simulink model "Modelo_DINAMICO_2021"  (R2021b)
settings: Solver=VariableStepAuto  StartTime=0.0  StopTime=0.1  MaxStep=1e-5  RelTol=1e-6
values from neighbouring files (symbols this model uses):
  AG0 = 10e-3    (= 0.01)    [Control_5GDL_V2_2021.m]
  beta = 20    [Control_5GDL_V2_2021.m]
  dTSensor = 5e-4    (= 0.0005)    [Control_5GDL_V2_2021.m]
  filterConstant = 30    [Control_5GDL_V2_2021.m]
  noiseSensor = 0.02*1e-3    (= 2e-05)    [Control_5GDL_V2_2021.m]
  z_0 = 17.5e-3    (= 0.0175)    [Control_5GDL_V2_2021.m]
  z_lev = pod.geometry.z_LEV    [Control_5GDL_V2_2021.m]
undefined symbols (not defined in the file or in its folder): initial_conds, pod
libraries: shared6dof x1, simulink_extras x1
settings Model: Creator=emate  LastModifiedBy=Ferran

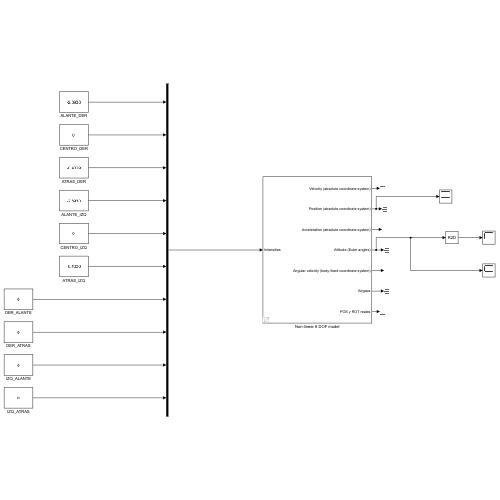
[thumbnail: Simulink's stored preview of the top-level diagram]
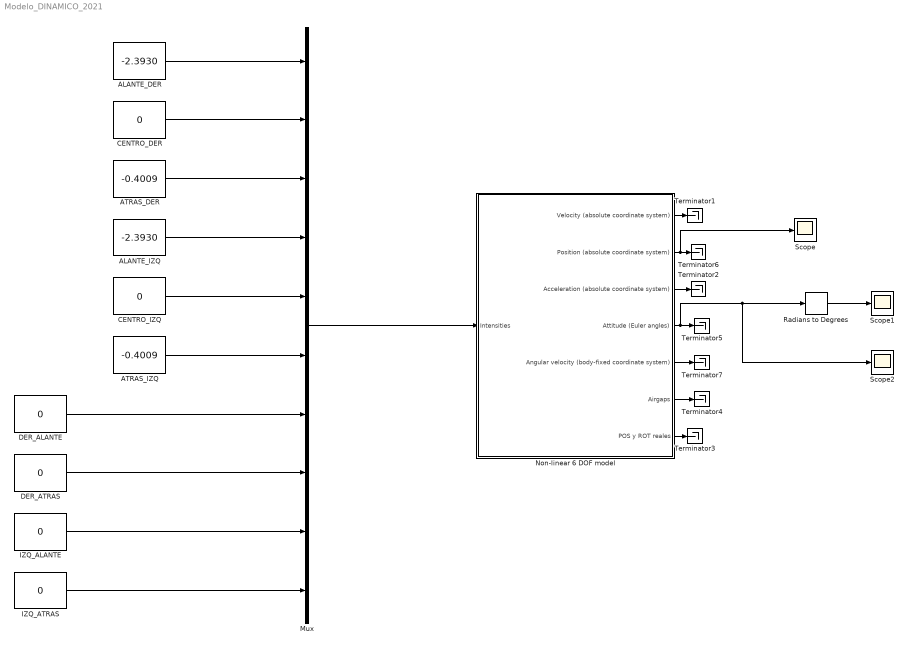
== system Modelo_DINAMICO_2021 ==
  ALANTE_DER : Constant  Value=-2.3930
  ALANTE_IZQ : Constant  Value=-2.3930
  ATRAS_DER : Constant  Value=-0.4009
  ATRAS_IZQ : Constant  Value=-0.4009
  CENTRO_DER : Constant  Value=0
  CENTRO_IZQ : Constant  Value=0
  DER_ALANTE : Constant  Value=0
  DER_ATRAS : Constant  Value=0
  IZQ_ALANTE : Constant  Value=0
  IZQ_ATRAS : Constant  Value=0
  Mux : Mux  Inputs=10
  Non-linear 6 DOF model : Subsystem  AncestorBlock=libH7_6DOF/Non-linear 6 DOF model
  Radians to Degrees : simulink_extras/Transformations/Radians to Degrees
  Scope : Scope
  Scope1 : Scope
  Scope2 : Scope
  Terminator{1..7} (7 alike) : Terminator
  wires:
  Mux/1 -> Non-linear 6 DOF model/1(Intensities)
  ALANTE_DER/1 -> Mux/1
  CENTRO_DER/1 -> Mux/2
  ATRAS_DER/1 -> Mux/3
  ALANTE_IZQ/1 -> Mux/4
  CENTRO_IZQ/1 -> Mux/5
  ATRAS_IZQ/1 -> Mux/6
  DER_ALANTE/1 -> Mux/7
  DER_ATRAS/1 -> Mux/8
  IZQ_ALANTE/1 -> Mux/9
  IZQ_ATRAS/1 -> Mux/10
  Non-linear 6 DOF model/1(Velocity (absolute coordinate system)) -> Terminator1/1
  Non-linear 6 DOF model/3(Acceleration (absolute coordinate system)) -> Terminator2/1
  Non-linear 6 DOF model/7(POS y ROT reales) -> Terminator3/1
  Non-linear 6 DOF model/6(Airgaps) -> Terminator4/1
  Non-linear 6 DOF model/2(Position (absolute coordinate system)) -> Scope/1, Terminator6/1
  Non-linear 6 DOF model/5(Angular velocity (body-fixed coordinate system)) -> Terminator7/1
  Non-linear 6 DOF model/4(Attitude (Euler angles)) -> Radians to Degrees/1, Scope2/1, Terminator5/1
  Radians to Degrees/1 -> Scope1/1

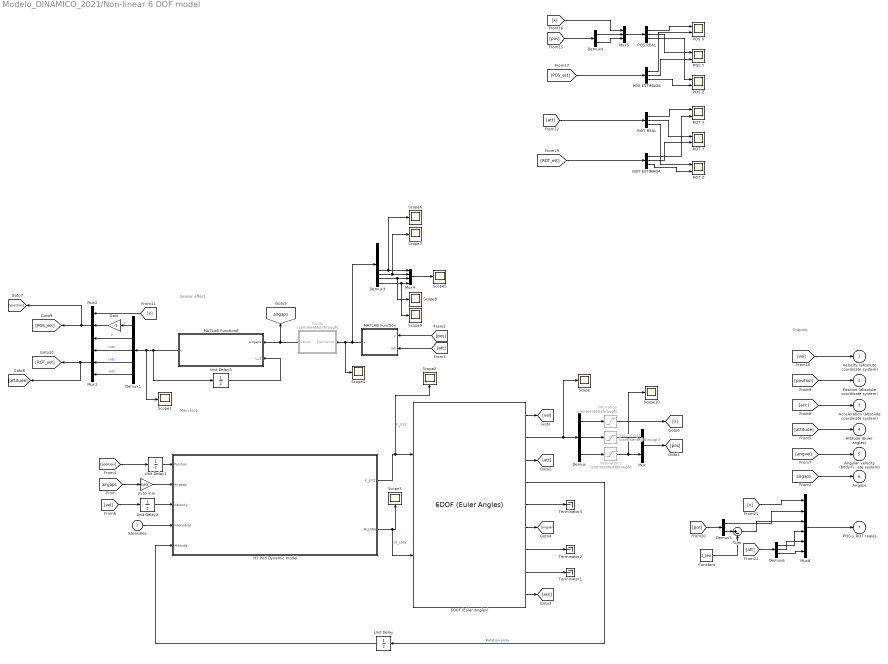
== system Modelo_DINAMICO_2021/Non-linear 6 DOF model ==
  note: Sensor effect
  note: Main loop
  note: Outputs
  Intensities : Inport
  " ROT X" : Scope  NumInputPorts=2
  " ROT Y" : Scope  NumInputPorts=2
  " ROT Z" : Scope  NumInputPorts=2
  6DOF (Euler Angles) : shared6dof/6DOF (Euler Angles)  units=Metric (MKS)  mtype=Fixed  rep=Euler Angles  xme_0=initial_conds.x_0  Vm_0=initial_conds.v_0  eul_0=initial_conds.ang_0  pm_0=initial_conds.w_0  mass_0=pod.mass.mass  mass_e=0.5  mass_f=2.0  inertia=pod.mass.inertia  inertia_e=eye(3)  inertia_f=2*eye(3)  k_quat=1.0  vre_flag=on  abi_flag=on  aMode=0  xme_statename=''  Vm_statename=''  eul_statename=''  quat_statename=''  pm_statename=''  mass_statename=''
      link override Abi: Port=9
      settings: SourceProductBaseCode=AE,PW,DR,MT,UV,VE
  Constant : Constant  Value=z_lev
  Demux : Demux  Outputs=3
  Demux1 : Demux  Outputs=5
  Demux3 : Demux  Outputs=10
  Demux4 : Demux  Outputs=2
  Demux5 : Demux  Outputs=2
  Demux6 : Demux  Outputs=3
  Gain : Gain  Gain=-1
  H7 Pod Dynamic model : Subsystem  AncestorBlock=libH7_6DOF/H7 Pod Dynamic model
      mask Display: image('FBD.png', [0.12 0.12 0.78 0.78]); % Use "Edit Image" on toolstrip to change.
  MATLAB Function : MATLAB Function  TreatAsAtomicUnit=on
  MATLAB Function2 : MATLAB Function  TreatAsAtomicUnit=on
  Mux : Mux  Inputs=2
  Mux1 : Mux  Inputs=3
  Mux2 : Mux  Inputs=3
  Mux4 : Mux
  Mux5 : Mux  Inputs=3
  Mux6 : Mux  Inputs=6
  POS ESTIMADA : Demux  Outputs=3
  POS REAL : Demux  Outputs=3
  POS X : Scope  NumInputPorts=2
  POS Y : Scope  NumInputPorts=2
  POS Z : Scope  NumInputPorts=2
  ROT ESTIMADA : Demux  Outputs=3
  ROT REAL : Demux  Outputs=3
  Ruido : Subsystem  Commented=through
  Saturation : Saturate  Commented=through  UpperLimit=20  LowerLimit=0
  Saturation1 : Saturate  Commented=through  UpperLimit=0.002  LowerLimit=-0.002
  Saturation2 : Saturate  Commented=through  UpperLimit=0.3504  LowerLimit=0.3384
  Scope{,1..10} (11 alike) : Scope
  Sum : Sum  Inputs=|+-
  Terminator1 : Terminator
  Terminator2 : Terminator
  Terminator3 : Terminator
  Unit Delay : UnitDelay  InitialCondition=eye(3,3)  SampleTime=-1  HasFrameUpgradeWarning=on
  Unit Delay1 : UnitDelay  InitialCondition=initial_conds.x_0  SampleTime=-1  HasFrameUpgradeWarning=on
  Unit Delay2 : UnitDelay  InitialCondition=initial_conds.v_0  SampleTime=-1  HasFrameUpgradeWarning=on
  Unit Delay3 : UnitDelay  SampleTime=-1  HasFrameUpgradeWarning=on
  m to mm : Gain  Gain=1e3
  Velocity (absolute coordinate system) : Outport
  Position (absolute coordinate system) : Outport  Port=2
  Acceleration (absolute coordinate system) : Outport  Port=3
  Attitude (Euler angles) : Outport  Port=4
  Angular velocity (body-fixed coordinate system) : Outport  Port=5
  Airgaps : Outport  Port=6
  POS y ROT reales : Outport  Port=7
  tag scope: airgaps=global
  wires:
  Demux1/3 -> Mux1/1  "rotx"
  6DOF (Euler Angles)/8 -> Terminator1/1
  6DOF (Euler Angles)/4 -> Unit Delay/1  "Rotation array"
  6DOF (Euler Angles)/7 -> Terminator2/1
  Unit Delay2/1 -> H7 Pod Dynamic model/3(Velocity)
  Demux/3 -> Saturation2/1
  H7 Pod Dynamic model/2(M_LMN) -> Scope3/1, 6DOF (Euler Angles)/2  "M_LMN"
  H7 Pod Dynamic model/1(F_XYZ) -> Scope2/1, 6DOF (Euler Angles)/1  "F_XYZ"
  Unit Delay/1 -> H7 Pod Dynamic model/5(Attitude)
  6DOF (Euler Angles)/3 -> [att]
  [airgaps] -> m to mm/1
  [position] -> Position (absolute coordinate system)/1
  [vel] -> Velocity (absolute coordinate system)/1
  [airgaps] -> Airgaps/1
  Unit Delay1/1 -> H7 Pod Dynamic model/1(Position)
  [angvel] -> Angular velocity (body-fixed coordinate system)/1
  6DOF (Euler Angles)/6 -> [angvel]
  6DOF (Euler Angles)/2 -> Scope/1, Demux/1
  Demux/2 -> Saturation1/1
  6DOF (Euler Angles)/9 -> [acc]
  [pos] -> MATLAB Function/1(r)
  MATLAB Function2/1(u) -> Unit Delay3/1, Scope1/1, Demux1/1
  [attitude] -> Attitude (Euler angles)/1
  Mux/1 -> [pos]
  Saturation/1 -> [x]
  [att] -> MATLAB Function/2(rot)
  Demux1/2 -> Mux2/3  "z"
  MATLAB Function/1(y) -> Demux3/1, Ruido/1(Estimation), Scope4/1
  Intensities/1 -> H7 Pod Dynamic model/4(Intensities)
  [position] -> Unit Delay1/1
  Unit Delay3/1 -> MATLAB Function2/2(u_1)
  6DOF (Euler Angles)/1 -> [vel]
  Demux1/4 -> Mux1/2  "roty"
  Demux1/5 -> Mux1/3  "rotz"
  [vel] -> Unit Delay2/1
  Demux/1 -> Saturation/1
  Ruido/1(Sensor) -> [airgaps], MATLAB Function2/1(airgaps)
  [x] -> Mux2/1
  Saturation1/1 -> Mux/1
  Demux1/1 -> Gain/1  "y"
  6DOF (Euler Angles)/5 -> Terminator3/1
  [acc] -> Acceleration (absolute coordinate system)/1
  Saturation2/1 -> Scope10/1, Mux/2
  m to mm/1 -> H7 Pod Dynamic model/2(Airgaps)
  Demux3/7 -> Scope6/1, Mux4/1
  Demux3/8 -> Scope7/1, Mux4/2
  Demux3/9 -> Scope8/1, Mux4/3
  Demux3/10 -> Scope9/1, Mux4/4
  Mux4/1 -> Scope5/1
  Mux2/1 -> [position], [POS_est]
  Mux1/1 -> [attitude], [ROT_est]
  [pos] -> Demux4/1
  [x] -> Mux5/1
  Demux4/1 -> Mux5/2
  Demux4/2 -> Mux5/3
  Mux5/1 -> POS REAL/1
  [POS_est] -> POS ESTIMADA/1
  POS REAL/1 -> POS X/1
  POS ESTIMADA/1 -> POS X/2
  POS REAL/2 -> POS Y/1
  POS ESTIMADA/2 -> POS Y/2
  POS ESTIMADA/3 -> POS Z/2
  POS REAL/3 -> POS Z/1
  [att] -> ROT REAL/1
  [ROT_est] -> ROT ESTIMADA/1
  ROT REAL/1 -> " ROT X"/1
  ROT ESTIMADA/1 -> " ROT X"/2
  ROT REAL/2 -> " ROT Y"/1
  ROT ESTIMADA/2 -> " ROT Y"/2
  ROT REAL/3 -> " ROT Z"/1
  ROT ESTIMADA/3 -> " ROT Z"/2
  Gain/1 -> Mux2/2
  [pos] -> Demux5/1
  [att] -> Demux6/1
  Mux6/1 -> POS y ROT reales/1
  [x] -> Mux6/1
  Demux5/1 -> Mux6/2
  Demux6/1 -> Mux6/4
  Demux6/2 -> Mux6/5
  Demux6/3 -> Mux6/6
  Demux5/2 -> Sum/1
  Sum/1 -> Mux6/3
  Constant/1 -> Sum/2

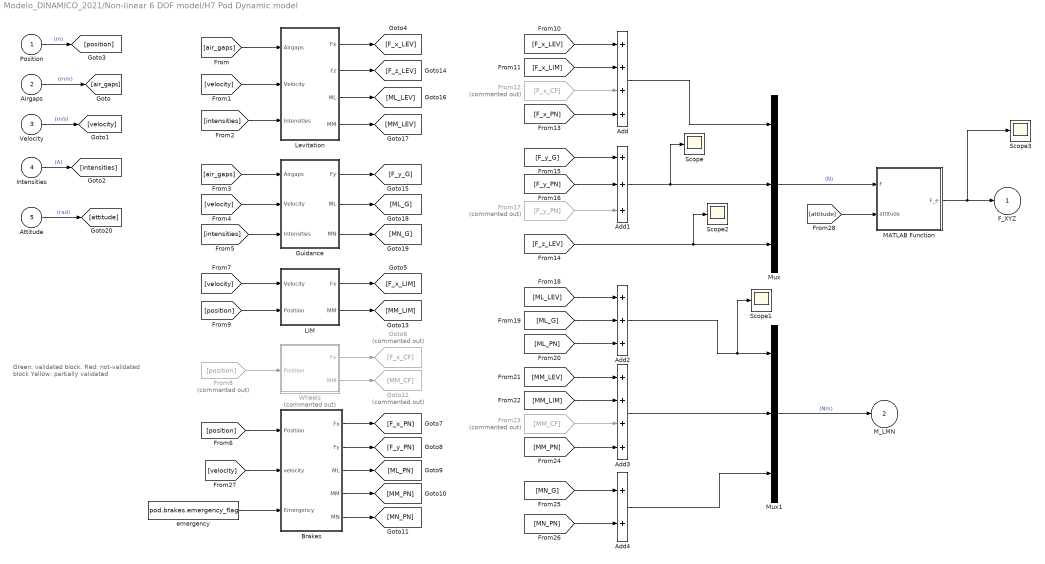
== system Modelo_DINAMICO_2021/Non-linear 6 DOF model/H7 Pod Dynamic model ==
  note: Green: validated block.
      | Red: not-validated block
      | Yellow: partially validated
  Position : Inport
  Airgaps : Inport  Port=2
  Velocity : Inport  Port=3
  Intensities : Inport  Port=4
  Attitude : Inport  Port=5
  Add : Sum  Inputs=++++
  Add1 : Sum  Inputs=+++
  Add2 : Sum  Inputs=+++
  Add3 : Sum  Inputs=++++
  Add4 : Sum
  Brakes : Subsystem
  From12 : From  Commented=on  GotoTag=F_x_CF
  From17 : From  Commented=on  GotoTag=F_y_PN
  From23 : From  Commented=on  GotoTag=MM_CF
  From8 : From  Commented=on  GotoTag=position
  Goto12 : Goto  Commented=on  GotoTag=MM_CF
  Goto6 : Goto  Commented=on  GotoTag=F_x_CF
  Guidance : Subsystem
  LIM : Subsystem
  Levitation : Subsystem
  MATLAB Function : MATLAB Function  TreatAsAtomicUnit=on
  Mux : Mux  Inputs=3
  Mux1 : Mux  Inputs=3
  Scope{,1..3} (4 alike) : Scope
  Wheels : Subsystem  Commented=on
  emergency : Constant  Value=pod.brakes.emergency_flag
  F_XYZ : Outport
  M_LMN : Outport  Port=2
  wires:
  Add3/1 -> Mux1/2
  [MM_LEV] -> Add3/1
  [MM_LIM] -> Add3/2
  [ML_LEV] -> Add2/1
  Add2/1 -> Scope1/1, Mux1/1
  [ML_G] -> Add2/2
  Add1/1 -> Scope/1, Mux/2
  [F_z_LEV] -> Scope2/1, Mux/3
  From12/1 -> Add/3
  [F_y_PN] -> Add1/2
  MATLAB Function/1(F_e) -> Scope3/1, F_XYZ/1
  Wheels/2(MM) -> Goto12/1
  [air_gaps] -> Levitation/1(Airgaps)
  Brakes/5(MN) -> [MN_PN]
  [F_x_LIM] -> Add/2
  Brakes/4(MM) -> [MM_PN]
  Levitation/2(Fz) -> [F_z_LEV]
  Guidance/3(MN) -> [MN_G]
  [F_x_LEV] -> Add/1
  Guidance/2(ML) -> [ML_G]
  Attitude/1 -> [attitude]  "(rad)"
  From17/1 -> Add1/3
  emergency/1 -> Brakes/3(Emergency)
  Add/1 -> Mux/1
  Add4/1 -> Mux1/3
  LIM/2(MM) -> [MM_LIM]
  [F_x_PN] -> Add/4
  Brakes/2(Fy) -> [F_y_PN]
  Levitation/4(MM) -> [MM_LEV]
  Wheels/1(Fx) -> Goto6/1
  Levitation/1(Fx) -> [F_x_LEV]
  [MM_PN] -> Add3/4
  Guidance/1(Fy) -> [F_y_G]
  From8/1 -> Wheels/1(Position)
  Brakes/1(Fx) -> [F_x_PN]
  Position/1 -> [position]  "(m)"
  [intensities] -> Levitation/3(Intensities)
  [position] -> Brakes/1(Position)
  [attitude] -> MATLAB Function/2(attitude)
  [position] -> LIM/2(Position)
  [MN_G] -> Add4/1
  [velocity] -> Brakes/2(velocity)
  [velocity] -> Levitation/2(Velocity)
  [MN_PN] -> Add4/2
  Levitation/3(ML) -> [ML_LEV]
  Brakes/3(ML) -> [ML_PN]
  [velocity] -> LIM/1(Velocity)
  LIM/1(Fx) -> [F_x_LIM]
  [air_gaps] -> Guidance/1(Airgaps)
  [intensities] -> Guidance/3(Intensities)
  Mux1/1 -> M_LMN/1  "(Nm)"
  [F_y_G] -> Add1/1
  From23/1 -> Add3/3
  [velocity] -> Guidance/2(Velocity)
  Mux/1 -> MATLAB Function/1(F)  "(N)"
  [ML_PN] -> Add2/3
  Intensities/1 -> [intensities]  "(A)"
  Velocity/1 -> [velocity]  "(m/s)"
  Airgaps/1 -> [air_gaps]  "(mm)"

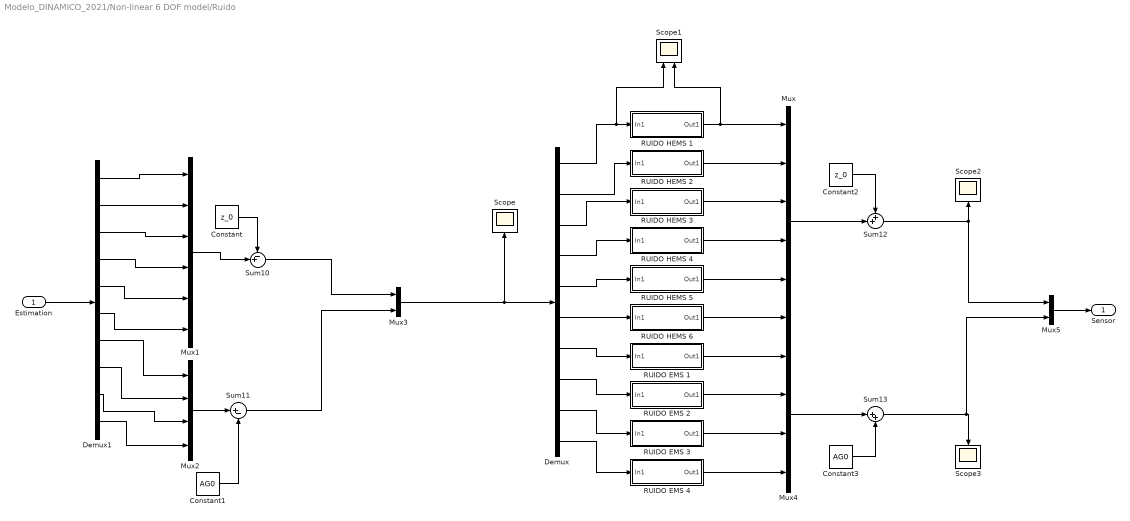
== system Modelo_DINAMICO_2021/Non-linear 6 DOF model/Ruido ==
  Estimation : Inport
  Constant : Constant  Value=z_0  SampleTime=dTSensor
  Constant1 : Constant  Value=AG0  SampleTime=dTSensor
  Constant2 : Constant  Value=z_0  SampleTime=dTSensor
  Constant3 : Constant  Value=AG0  SampleTime=dTSensor
  Demux : Demux  Outputs=10
  Demux1 : Demux  Outputs=10
  Mux : Mux  Inputs=6
  Mux1 : Mux  Inputs=6
  Mux2 : Mux
  Mux3 : Mux  Inputs=2
  Mux4 : Mux
  Mux5 : Mux  Inputs=2
  RUIDO EMS 1 : Subsystem
  RUIDO EMS 2 : Subsystem
  RUIDO EMS 3 : Subsystem
  RUIDO EMS 4 : Subsystem
  RUIDO HEMS 1 : Subsystem
  RUIDO HEMS 2 : Subsystem
  RUIDO HEMS 3 : Subsystem
  RUIDO HEMS 4 : Subsystem
  RUIDO HEMS 5 : Subsystem
  RUIDO HEMS 6 : Subsystem
  Scope : Scope
  Scope1 : Scope  NumInputPorts=2
  Scope2 : Scope
  Scope3 : Scope
  Sum10 : Sum  Inputs=-+|
  Sum11 : Sum  Inputs=|+-
  Sum12 : Sum  Inputs=++|
  Sum13 : Sum  Inputs=|++
  Sensor : Outport
  wires:
  Demux1/5 -> Mux1/5
  Mux3/1 -> Demux/1, Scope/1
  Demux1/6 -> Mux1/6
  Sum10/1 -> Mux3/1
  Constant1/1 -> Sum11/2
  Mux2/1 -> Sum11/1
  Demux1/10 -> Mux2/4
  Demux1/2 -> Mux1/2
  Constant/1 -> Sum10/1
  Demux1/7 -> Mux2/1
  Mux1/1 -> Sum10/2
  Demux1/8 -> Mux2/2
  Estimation/1 -> Demux1/1
  Demux1/4 -> Mux1/4
  Demux1/3 -> Mux1/3
  Demux1/1 -> Mux1/1
  Demux1/9 -> Mux2/3
  Sum11/1 -> Mux3/2
  Demux/2 -> RUIDO HEMS 2/1(In1)
  Demux/3 -> RUIDO HEMS 3/1(In1)
  Demux/4 -> RUIDO HEMS 4/1(In1)
  Demux/5 -> RUIDO HEMS 5/1(In1)
  Demux/6 -> RUIDO HEMS 6/1(In1)
  Demux/7 -> RUIDO EMS 1/1(In1)
  Demux/8 -> RUIDO EMS 2/1(In1)
  Demux/9 -> RUIDO EMS 3/1(In1)
  Demux/10 -> RUIDO EMS 4/1(In1)
  RUIDO HEMS 1/1(Out1) -> Scope1/2, Mux/1
  RUIDO HEMS 2/1(Out1) -> Mux/2
  RUIDO HEMS 3/1(Out1) -> Mux/3
  RUIDO HEMS 4/1(Out1) -> Mux/4
  RUIDO HEMS 5/1(Out1) -> Mux/5
  RUIDO HEMS 6/1(Out1) -> Mux/6
  RUIDO EMS 1/1(Out1) -> Mux4/1
  RUIDO EMS 2/1(Out1) -> Mux4/2
  RUIDO EMS 3/1(Out1) -> Mux4/3
  RUIDO EMS 4/1(Out1) -> Mux4/4
  Constant2/1 -> Sum12/1
  Mux/1 -> Sum12/2
  Sum13/1 -> Mux5/2, Scope3/1
  Constant3/1 -> Sum13/2
  Mux4/1 -> Sum13/1
  Sum12/1 -> Mux5/1, Scope2/1
  Mux5/1 -> Sensor/1
  Demux/1 -> Scope1/1, RUIDO HEMS 1/1(In1)

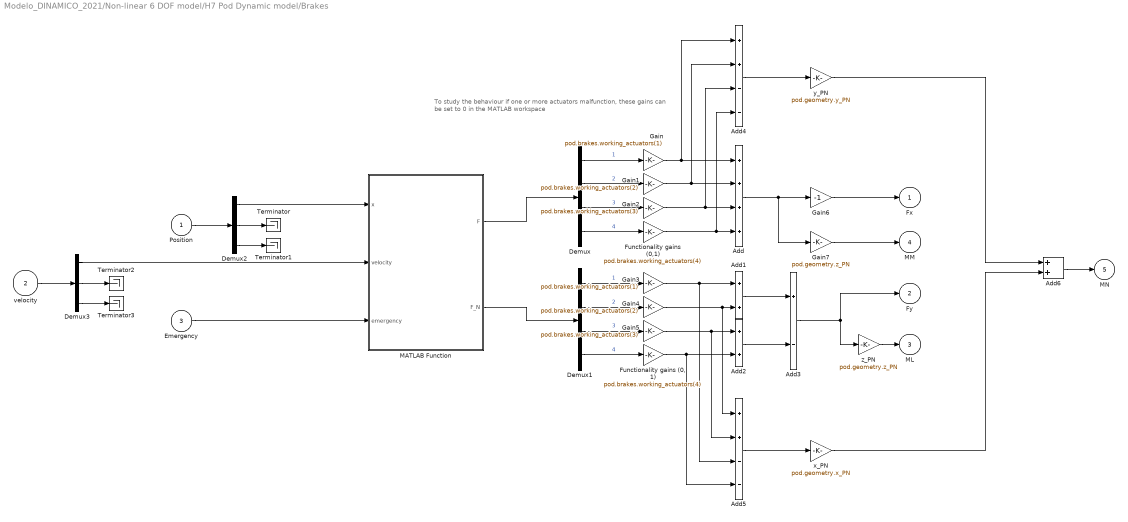
== system Modelo_DINAMICO_2021/Non-linear 6 DOF model/H7 Pod Dynamic model/Brakes ==
  note: To study the behaviour if one or more actuators malfunction,
      | these gains can be set to 0 in the MATLAB workspace
  Position : Inport
  velocity : Inport  Port=2
  Emergency : Inport  Port=3
  Add : Sum  Inputs=++++
  Add1 : Sum
  Add2 : Sum
  Add3 : Sum  Inputs=+-
  Add4 : Sum  Inputs=++--
  Add5 : Sum  Inputs=++--
  Add6 : Sum
  Demux : Demux
  Demux1 : Demux
  Demux2 : Demux  Outputs=3
  Demux3 : Demux  Outputs=3
  "Functionality gains (0, 1)" : Gain  Gain=pod.brakes.working_actuators(4)
  Functionality gains (0,1) : Gain  Gain=pod.brakes.working_actuators(4)
  Gain : Gain  Gain=pod.brakes.working_actuators(1)
  Gain1 : Gain  Gain=pod.brakes.working_actuators(2)
  Gain2 : Gain  Gain=pod.brakes.working_actuators(3)
  Gain3 : Gain  Gain=pod.brakes.working_actuators(1)
  Gain4 : Gain  Gain=pod.brakes.working_actuators(2)
  Gain5 : Gain  Gain=pod.brakes.working_actuators(3)
  Gain6 : Gain  Gain=-1
  Gain7 : Gain  Gain=pod.geometry.z_PN
  MATLAB Function : MATLAB Function  TreatAsAtomicUnit=on
  Terminator{,1..3} (4 alike) : Terminator
  x_PN : Gain  Gain=pod.geometry.x_PN
  y_PN : Gain  Gain=pod.geometry.y_PN
  z_PN : Gain  Gain=pod.geometry.z_PN
  Fx : Outport
  Fy : Outport  Port=2
  ML : Outport  Port=3
  MM : Outport  Port=4
  MN : Outport  Port=5
  wires:
  Emergency/1 -> MATLAB Function/3(emergency)
  MATLAB Function/1(F) -> Demux/1
  Demux/1 -> Gain/1  "1"
  Demux/2 -> Gain1/1  "2"
  Demux/3 -> Gain2/1  "3"
  Demux/4 -> Functionality gains (0,1)/1  "4"
  Demux1/4 -> "Functionality gains (0, 1)"/1  "4"
  Demux1/3 -> Gain5/1  "3"
  Demux1/1 -> Gain3/1  "1"
  Demux1/2 -> Gain4/1  "2"
  MATLAB Function/2(F_N) -> Demux1/1
  Functionality gains (0,1)/1 -> Add4/4, Add/4
  Gain2/1 -> Add4/3, Add/3
  Gain1/1 -> Add4/2, Add/2
  Gain/1 -> Add4/1, Add/1
  Add/1 -> Gain7/1, Gain6/1
  Gain6/1 -> Fx/1
  Gain4/1 -> Add5/1, Add1/2
  Gain3/1 -> Add1/1, Add5/3
  Gain5/1 -> Add5/2, Add2/1
  "Functionality gains (0, 1)"/1 -> Add2/2, Add5/4
  Add1/1 -> Add3/1
  Add2/1 -> Add3/2
  Add3/1 -> z_PN/1, Fy/1
  z_PN/1 -> ML/1
  Gain7/1 -> MM/1
  Add4/1 -> y_PN/1
  Demux2/3 -> Terminator1/1
  Position/1 -> Demux2/1
  Demux2/1 -> MATLAB Function/1(x)
  Demux2/2 -> Terminator/1
  velocity/1 -> Demux3/1
  Demux3/2 -> Terminator2/1
  Demux3/3 -> Terminator3/1
  Demux3/1 -> MATLAB Function/2(velocity)
  Add5/1 -> x_PN/1
  Add6/1 -> MN/1
  y_PN/1 -> Add6/1
  x_PN/1 -> Add6/2

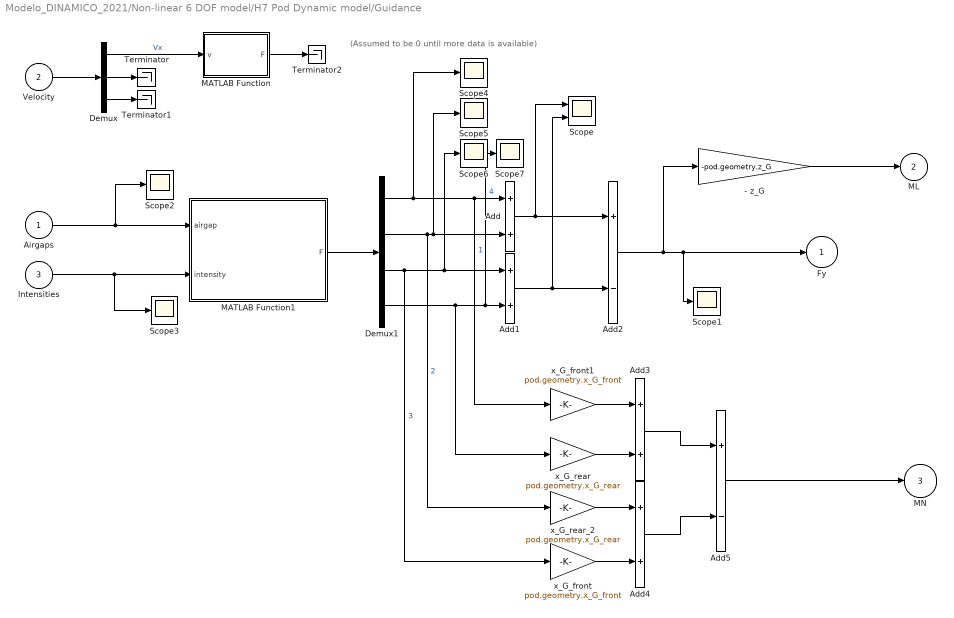
== system Modelo_DINAMICO_2021/Non-linear 6 DOF model/H7 Pod Dynamic model/Guidance ==
  note: (Assumed to be 0 until more data is available)
  Airgaps : Inport
  Velocity : Inport  Port=2
  Intensities : Inport  Port=3
  " x_G_front" : Gain  Gain=pod.geometry.x_G_front
  " x_G_front1" : Gain  Gain=pod.geometry.x_G_front
  " x_G_rear" : Gain  Gain=pod.geometry.x_G_rear
  " x_G_rear_2" : Gain  Gain=pod.geometry.x_G_rear
  - z_G : Gain  Gain=-pod.geometry.z_G
  Add{,1,3..4} (4 alike) : Sum
  Add2 : Sum  Inputs=+-
  Add5 : Sum  Inputs=+-
  Demux : Demux  Outputs=3
  Demux1 : Demux
  MATLAB Function : MATLAB Function  TreatAsAtomicUnit=on
  MATLAB Function1 : MATLAB Function  TreatAsAtomicUnit=on
  Scope : Scope  NumInputPorts=2
  Scope{1..7} (7 alike) : Scope
  Terminator : Terminator
  Terminator1 : Terminator
  Terminator2 : Terminator
  Fy : Outport
  ML : Outport  Port=2
  MN : Outport  Port=3
  wires:
  Demux/1 -> MATLAB Function/1(v)  "Vx"
  Velocity/1 -> Demux/1
  Demux/2 -> Terminator/1
  Demux/3 -> Terminator1/1
  MATLAB Function/1(F) -> Terminator2/1
  Intensities/1 -> Scope3/1, MATLAB Function1/2(intensity)
  Airgaps/1 -> Scope2/1, MATLAB Function1/1(airgap)
  Demux1/1 -> Scope4/1, " x_G_front1"/1, Add/1  "1"
  Demux1/2 -> " x_G_rear_2"/1, Scope5/1, Add/2  "2"
  Demux1/3 -> " x_G_front"/1, Scope6/1, Add1/1  "3"
  Demux1/4 -> " x_G_rear"/1, Scope7/1, Add1/2  "4"
  Add1/1 -> Scope/2, Add2/2
  Add/1 -> Scope/1, Add2/1
  Add2/1 -> - z_G/1, Scope1/1, Fy/1
  - z_G/1 -> ML/1
  Add3/1 -> Add5/1
  Add4/1 -> Add5/2
  Add5/1 -> MN/1
  MATLAB Function1/1(F) -> Demux1/1
  " x_G_front"/1 -> Add4/2
  " x_G_front1"/1 -> Add3/1
  " x_G_rear"/1 -> Add3/2
  " x_G_rear_2"/1 -> Add4/1

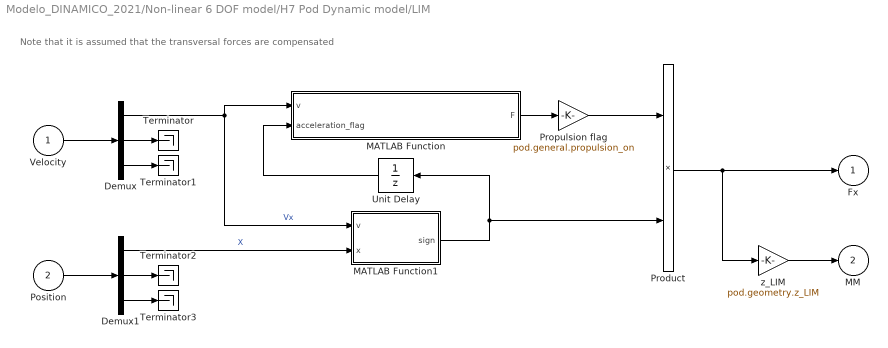
== system Modelo_DINAMICO_2021/Non-linear 6 DOF model/H7 Pod Dynamic model/LIM ==
  note: Note that it is assumed that the transversal forces are compensated
  Velocity : Inport
  Position : Inport  Port=2
  Demux : Demux  Outputs=3
  Demux1 : Demux  Outputs=3
  MATLAB Function : MATLAB Function  TreatAsAtomicUnit=on
  MATLAB Function1 : MATLAB Function  TreatAsAtomicUnit=on
  Product : Product
  Propulsion flag : Gain  Gain=pod.general.propulsion_on
  Terminator{,1..3} (4 alike) : Terminator
  Unit Delay : UnitDelay  InitialCondition=1  SampleTime=-1  HasFrameUpgradeWarning=on
  z_LIM : Gain  Gain=pod.geometry.z_LIM
  Fx : Outport
  MM : Outport  Port=2
  wires:
  Unit Delay/1 -> MATLAB Function/2(acceleration_flag)
  Propulsion flag/1 -> Product/1
  Velocity/1 -> Demux/1
  Demux/2 -> Terminator/1
  Demux/3 -> Terminator1/1
  Demux/1 -> MATLAB Function1/1(v), MATLAB Function/1(v)  "Vx"
  Position/1 -> Demux1/1
  Demux1/3 -> Terminator3/1
  Demux1/2 -> Terminator2/1
  Demux1/1 -> MATLAB Function1/2(x)  "X"
  MATLAB Function1/1(sign) -> Product/2, Unit Delay/1
  MATLAB Function/1(F) -> Propulsion flag/1
  Product/1 -> z_LIM/1, Fx/1
  z_LIM/1 -> MM/1

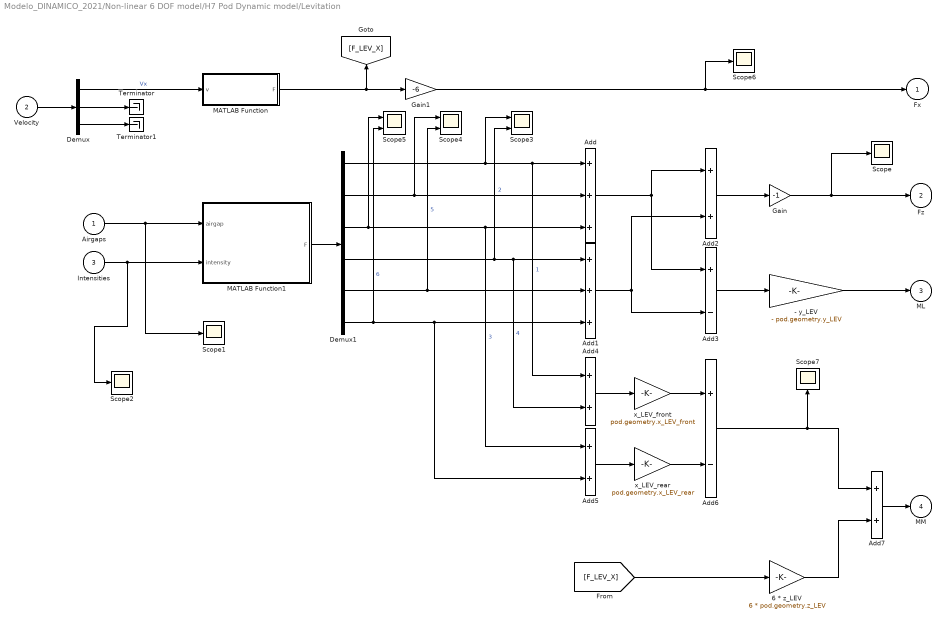
== system Modelo_DINAMICO_2021/Non-linear 6 DOF model/H7 Pod Dynamic model/Levitation ==
  Airgaps : Inport
  Velocity : Inport  Port=2
  Intensities : Inport  Port=3
  - y_LEV : Gain  Gain=- pod.geometry.y_LEV
  6 * z_LEV : Gain  Gain=6 * pod.geometry.z_LEV
  Add : Sum  Inputs=+++
  Add1 : Sum  Inputs=+++
  Add{2,4..5,7} (4 alike) : Sum
  Add3 : Sum  Inputs=+-
  Add6 : Sum  Inputs=+-
  Demux : Demux  Outputs=3
  Demux1 : Demux  Outputs=6
  Gain : Gain  Gain=-1
  Gain1 : Gain  Gain=-6
  MATLAB Function : MATLAB Function  TreatAsAtomicUnit=on
  MATLAB Function1 : MATLAB Function  TreatAsAtomicUnit=on
  Scope{,1..2,6..7} (5 alike) : Scope
  Scope3 : Scope  NumInputPorts=2
  Scope4 : Scope  NumInputPorts=2
  Scope5 : Scope  NumInputPorts=2
  Terminator : Terminator
  Terminator1 : Terminator
  x_LEV_front : Gain  Gain=pod.geometry.x_LEV_front
  x_LEV_rear : Gain  Gain=pod.geometry.x_LEV_rear
  Fx : Outport
  Fz : Outport  Port=2
  ML : Outport  Port=3
  MM : Outport  Port=4
  wires:
  Demux/2 -> Terminator/1
  Demux/3 -> Terminator1/1
  Velocity/1 -> Demux/1
  Demux/1 -> MATLAB Function/1(v)  "Vx"
  Airgaps/1 -> MATLAB Function1/1(airgap), Scope1/1
  Intensities/1 -> MATLAB Function1/2(intensity), Scope2/1
  MATLAB Function1/1(F) -> Demux1/1
  Gain/1 -> Fz/1, Scope/1
  Demux1/1 -> Scope3/1, Add4/1, Add/1  "1"
  Demux1/2 -> Scope4/1, Add/2  "2"
  Demux1/3 -> Scope5/1, Add5/1, Add/3  "3"
  Demux1/4 -> Scope3/2, Add4/2, Add1/1  "4"
  Demux1/5 -> Add1/2, Scope4/2  "5"
  Demux1/6 -> Scope5/2, Add5/2, Add1/3  "6"
  Add/1 -> Add2/1, Add3/1
  Add1/1 -> Add2/2, Add3/2
  Add2/1 -> Gain/1
  Add3/1 -> - y_LEV/1
  - y_LEV/1 -> ML/1
  Gain1/1 -> Scope6/1, Fx/1
  [F_LEV_X] -> 6 * z_LEV/1
  Add4/1 -> x_LEV_front/1
  Add5/1 -> x_LEV_rear/1
  Add7/1 -> MM/1
  Add6/1 -> Scope7/1, Add7/1
  6 * z_LEV/1 -> Add7/2
  MATLAB Function/1(F) -> [F_LEV_X], Gain1/1
  x_LEV_front/1 -> Add6/1
  x_LEV_rear/1 -> Add6/2

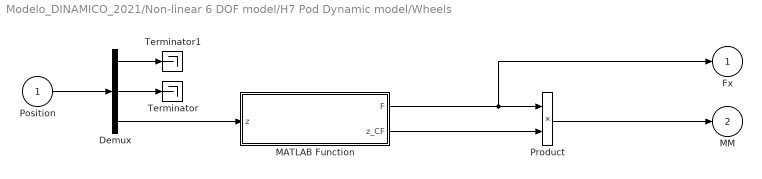
== system Modelo_DINAMICO_2021/Non-linear 6 DOF model/H7 Pod Dynamic model/Wheels ==
  Position : Inport
  Demux : Demux  Outputs=3
  MATLAB Function : MATLAB Function  TreatAsAtomicUnit=on
  Product : Product
  Terminator : Terminator
  Terminator1 : Terminator
  Fx : Outport
  MM : Outport  Port=2
  wires:
  Position/1 -> Demux/1
  Demux/2 -> Terminator/1
  Demux/3 -> MATLAB Function/1(z)
  MATLAB Function/1(F) -> Fx/1, Product/1
  Demux/1 -> Terminator1/1
  MATLAB Function/2(z_CF) -> Product/2
  Product/1 -> MM/1

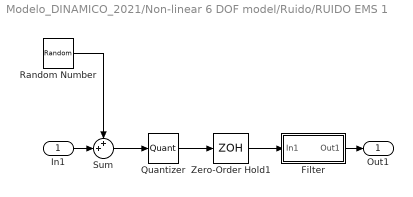
== system Modelo_DINAMICO_2021/Non-linear 6 DOF model/Ruido/RUIDO EMS 1 ==
  In1 : Inport
  Filter : Subsystem
  Quantizer : Quantizer  QuantizationInterval=resSensor
  Random Number : RandomNumber  Variance=noiseSensor^2  Seed=24
  Sum : Sum  Inputs=++|
  Zero-Order Hold1 : ZeroOrderHold  SampleTime=dTSensor
  Out1 : Outport
  wires:
  Random Number/1 -> Sum/1
  Zero-Order Hold1/1 -> Filter/1(In1)
  In1/1 -> Sum/2
  Sum/1 -> Quantizer/1
  Quantizer/1 -> Zero-Order Hold1/1
  Filter/1(Out1) -> Out1/1

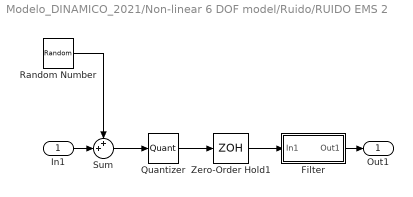
== system Modelo_DINAMICO_2021/Non-linear 6 DOF model/Ruido/RUIDO EMS 2 ==
  In1 : Inport
  Filter : Subsystem
  Quantizer : Quantizer  QuantizationInterval=resSensor
  Random Number : RandomNumber  Variance=noiseSensor^2  Seed=27
  Sum : Sum  Inputs=++|
  Zero-Order Hold1 : ZeroOrderHold  SampleTime=dTSensor
  Out1 : Outport
  wires:
  Filter/1(Out1) -> Out1/1
  Quantizer/1 -> Zero-Order Hold1/1
  Sum/1 -> Quantizer/1
  In1/1 -> Sum/2
  Zero-Order Hold1/1 -> Filter/1(In1)
  Random Number/1 -> Sum/1

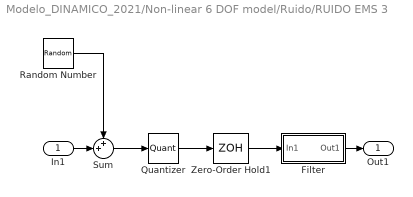
== system Modelo_DINAMICO_2021/Non-linear 6 DOF model/Ruido/RUIDO EMS 3 ==
  In1 : Inport
  Filter : Subsystem
  Quantizer : Quantizer  QuantizationInterval=resSensor
  Random Number : RandomNumber  Variance=noiseSensor^2  Seed=29
  Sum : Sum  Inputs=++|
  Zero-Order Hold1 : ZeroOrderHold  SampleTime=dTSensor
  Out1 : Outport
  wires:
  Random Number/1 -> Sum/1
  Zero-Order Hold1/1 -> Filter/1(In1)
  In1/1 -> Sum/2
  Sum/1 -> Quantizer/1
  Quantizer/1 -> Zero-Order Hold1/1
  Filter/1(Out1) -> Out1/1

== system Modelo_DINAMICO_2021/Non-linear 6 DOF model/Ruido/RUIDO EMS 4 ==
  In1 : Inport
  Filter : Subsystem
  Quantizer : Quantizer  QuantizationInterval=resSensor
  Random Number : RandomNumber  Variance=noiseSensor^2  Seed=30
  Sum : Sum  Inputs=++|
  Zero-Order Hold1 : ZeroOrderHold  SampleTime=dTSensor
  Out1 : Outport
  wires:
  Filter/1(Out1) -> Out1/1
  Quantizer/1 -> Zero-Order Hold1/1
  Sum/1 -> Quantizer/1
  In1/1 -> Sum/2
  Zero-Order Hold1/1 -> Filter/1(In1)
  Random Number/1 -> Sum/1

== system Modelo_DINAMICO_2021/Non-linear 6 DOF model/Ruido/RUIDO HEMS 1 ==
  In1 : Inport
  Filter : Subsystem
  Quantizer : Quantizer  QuantizationInterval=resSensor
  Random Number : RandomNumber  Variance=noiseSensor^2  Seed=14
  Sum : Sum  Inputs=++|
  Zero-Order Hold1 : ZeroOrderHold  SampleTime=dTSensor
  Out1 : Outport
  wires:
  Random Number/1 -> Sum/1
  Zero-Order Hold1/1 -> Filter/1(In1)
  In1/1 -> Sum/2
  Sum/1 -> Quantizer/1
  Quantizer/1 -> Zero-Order Hold1/1
  Filter/1(Out1) -> Out1/1

== system Modelo_DINAMICO_2021/Non-linear 6 DOF model/Ruido/RUIDO HEMS 2 ==
  In1 : Inport
  Filter : Subsystem
  Quantizer : Quantizer  QuantizationInterval=resSensor
  Random Number : RandomNumber  Variance=noiseSensor^2  Seed=1
  Sum : Sum  Inputs=++|
  Zero-Order Hold1 : ZeroOrderHold  SampleTime=dTSensor
  Out1 : Outport
  wires:
  Filter/1(Out1) -> Out1/1
  Quantizer/1 -> Zero-Order Hold1/1
  Sum/1 -> Quantizer/1
  In1/1 -> Sum/2
  Zero-Order Hold1/1 -> Filter/1(In1)
  Random Number/1 -> Sum/1

== system Modelo_DINAMICO_2021/Non-linear 6 DOF model/Ruido/RUIDO HEMS 3 ==
  In1 : Inport
  Filter : Subsystem
  Quantizer : Quantizer  QuantizationInterval=resSensor
  Random Number : RandomNumber  Variance=noiseSensor^2  Seed=3
  Sum : Sum  Inputs=++|
  Zero-Order Hold1 : ZeroOrderHold  SampleTime=dTSensor
  Out1 : Outport
  wires:
  Random Number/1 -> Sum/1
  Zero-Order Hold1/1 -> Filter/1(In1)
  In1/1 -> Sum/2
  Sum/1 -> Quantizer/1
  Quantizer/1 -> Zero-Order Hold1/1
  Filter/1(Out1) -> Out1/1

== system Modelo_DINAMICO_2021/Non-linear 6 DOF model/Ruido/RUIDO HEMS 4 ==
  In1 : Inport
  Filter : Subsystem
  Quantizer : Quantizer  QuantizationInterval=resSensor
  Random Number : RandomNumber  Variance=noiseSensor^2  Seed=7
  Sum : Sum  Inputs=++|
  Zero-Order Hold1 : ZeroOrderHold  SampleTime=dTSensor
  Out1 : Outport
  wires:
  Filter/1(Out1) -> Out1/1
  Quantizer/1 -> Zero-Order Hold1/1
  Sum/1 -> Quantizer/1
  In1/1 -> Sum/2
  Zero-Order Hold1/1 -> Filter/1(In1)
  Random Number/1 -> Sum/1

== system Modelo_DINAMICO_2021/Non-linear 6 DOF model/Ruido/RUIDO HEMS 5 ==
  In1 : Inport
  Filter : Subsystem
  Quantizer : Quantizer  QuantizationInterval=resSensor
  Random Number : RandomNumber  Variance=noiseSensor^2  Seed=11
  Sum : Sum  Inputs=++|
  Zero-Order Hold1 : ZeroOrderHold  SampleTime=dTSensor
  Out1 : Outport
  wires:
  Random Number/1 -> Sum/1
  Zero-Order Hold1/1 -> Filter/1(In1)
  In1/1 -> Sum/2
  Sum/1 -> Quantizer/1
  Quantizer/1 -> Zero-Order Hold1/1
  Filter/1(Out1) -> Out1/1

== system Modelo_DINAMICO_2021/Non-linear 6 DOF model/Ruido/RUIDO HEMS 6 ==
  In1 : Inport
  Filter : Subsystem
  Quantizer : Quantizer  QuantizationInterval=resSensor
  Random Number : RandomNumber  Variance=noiseSensor^2  Seed=21
  Sum : Sum  Inputs=++|
  Zero-Order Hold1 : ZeroOrderHold  SampleTime=dTSensor
  Out1 : Outport
  wires:
  Filter/1(Out1) -> Out1/1
  Quantizer/1 -> Zero-Order Hold1/1
  Sum/1 -> Quantizer/1
  In1/1 -> Sum/2
  Zero-Order Hold1/1 -> Filter/1(In1)
  Random Number/1 -> Sum/1

== system Modelo_DINAMICO_2021/Non-linear 6 DOF model/Ruido/RUIDO EMS 1/Filter ==
  In1 : Inport
  Gain : Gain  Gain=filterConstant
  Gain1 : Gain  Gain=1/(filterConstant+1)
  Sum : Sum  Inputs=|++
  Unit Delay : UnitDelay  SampleTime=dTSensor  HasFrameUpgradeWarning=on
  Out1 : Outport
  wires:
  Gain/1 -> Sum/2
  Sum/1 -> Gain1/1
  Gain1/1 -> Out1/1, Unit Delay/1
  Unit Delay/1 -> Gain/1
  In1/1 -> Sum/1

== system Modelo_DINAMICO_2021/Non-linear 6 DOF model/Ruido/RUIDO EMS 2/Filter ==
  In1 : Inport
  Gain : Gain  Gain=filterConstant
  Gain1 : Gain  Gain=1/(filterConstant+1)
  Sum : Sum  Inputs=|++
  Unit Delay : UnitDelay  SampleTime=dTSensor  HasFrameUpgradeWarning=on
  Out1 : Outport
  wires:
  In1/1 -> Sum/1
  Unit Delay/1 -> Gain/1
  Gain1/1 -> Unit Delay/1, Out1/1
  Sum/1 -> Gain1/1
  Gain/1 -> Sum/2

== system Modelo_DINAMICO_2021/Non-linear 6 DOF model/Ruido/RUIDO EMS 3/Filter ==
  In1 : Inport
  Gain : Gain  Gain=filterConstant
  Gain1 : Gain  Gain=1/(filterConstant+1)
  Sum : Sum  Inputs=|++
  Unit Delay : UnitDelay  SampleTime=dTSensor  HasFrameUpgradeWarning=on
  Out1 : Outport
  wires:
  Gain/1 -> Sum/2
  Sum/1 -> Gain1/1
  Gain1/1 -> Out1/1, Unit Delay/1
  Unit Delay/1 -> Gain/1
  In1/1 -> Sum/1

== system Modelo_DINAMICO_2021/Non-linear 6 DOF model/Ruido/RUIDO EMS 4/Filter ==
  In1 : Inport
  Gain : Gain  Gain=filterConstant
  Gain1 : Gain  Gain=1/(filterConstant+1)
  Sum : Sum  Inputs=|++
  Unit Delay : UnitDelay  SampleTime=dTSensor  HasFrameUpgradeWarning=on
  Out1 : Outport
  wires:
  In1/1 -> Sum/1
  Unit Delay/1 -> Gain/1
  Gain1/1 -> Unit Delay/1, Out1/1
  Sum/1 -> Gain1/1
  Gain/1 -> Sum/2

== system Modelo_DINAMICO_2021/Non-linear 6 DOF model/Ruido/RUIDO HEMS 1/Filter ==
  In1 : Inport
  Gain : Gain  Gain=filterConstant
  Gain1 : Gain  Gain=1/(filterConstant+1)
  Sum : Sum  Inputs=|++
  Unit Delay : UnitDelay  SampleTime=dTSensor  HasFrameUpgradeWarning=on
  Out1 : Outport
  wires:
  Gain/1 -> Sum/2
  Sum/1 -> Gain1/1
  Gain1/1 -> Out1/1, Unit Delay/1
  Unit Delay/1 -> Gain/1
  In1/1 -> Sum/1

== system Modelo_DINAMICO_2021/Non-linear 6 DOF model/Ruido/RUIDO HEMS 2/Filter ==
  In1 : Inport
  Gain : Gain  Gain=filterConstant
  Gain1 : Gain  Gain=1/(filterConstant+1)
  Sum : Sum  Inputs=|++
  Unit Delay : UnitDelay  SampleTime=dTSensor  HasFrameUpgradeWarning=on
  Out1 : Outport
  wires:
  In1/1 -> Sum/1
  Unit Delay/1 -> Gain/1
  Gain1/1 -> Unit Delay/1, Out1/1
  Sum/1 -> Gain1/1
  Gain/1 -> Sum/2

== system Modelo_DINAMICO_2021/Non-linear 6 DOF model/Ruido/RUIDO HEMS 3/Filter ==
  In1 : Inport
  Gain : Gain  Gain=filterConstant
  Gain1 : Gain  Gain=1/(filterConstant+1)
  Sum : Sum  Inputs=|++
  Unit Delay : UnitDelay  SampleTime=dTSensor  HasFrameUpgradeWarning=on
  Out1 : Outport
  wires:
  Gain/1 -> Sum/2
  Sum/1 -> Gain1/1
  Gain1/1 -> Out1/1, Unit Delay/1
  Unit Delay/1 -> Gain/1
  In1/1 -> Sum/1

== system Modelo_DINAMICO_2021/Non-linear 6 DOF model/Ruido/RUIDO HEMS 4/Filter ==
  In1 : Inport
  Gain : Gain  Gain=filterConstant
  Gain1 : Gain  Gain=1/(filterConstant+1)
  Sum : Sum  Inputs=|++
  Unit Delay : UnitDelay  SampleTime=dTSensor  HasFrameUpgradeWarning=on
  Out1 : Outport
  wires:
  In1/1 -> Sum/1
  Unit Delay/1 -> Gain/1
  Gain1/1 -> Unit Delay/1, Out1/1
  Sum/1 -> Gain1/1
  Gain/1 -> Sum/2

== system Modelo_DINAMICO_2021/Non-linear 6 DOF model/Ruido/RUIDO HEMS 5/Filter ==
  In1 : Inport
  Gain : Gain  Gain=filterConstant
  Gain1 : Gain  Gain=1/(filterConstant+1)
  Sum : Sum  Inputs=|++
  Unit Delay : UnitDelay  SampleTime=dTSensor  HasFrameUpgradeWarning=on
  Out1 : Outport
  wires:
  Gain/1 -> Sum/2
  Sum/1 -> Gain1/1
  Gain1/1 -> Out1/1, Unit Delay/1
  Unit Delay/1 -> Gain/1
  In1/1 -> Sum/1

== system Modelo_DINAMICO_2021/Non-linear 6 DOF model/Ruido/RUIDO HEMS 6/Filter ==
  In1 : Inport
  Gain : Gain  Gain=filterConstant
  Gain1 : Gain  Gain=1/(filterConstant+1)
  Sum : Sum  Inputs=|++
  Unit Delay : UnitDelay  SampleTime=dTSensor  HasFrameUpgradeWarning=on
  Out1 : Outport
  wires:
  In1/1 -> Sum/1
  Unit Delay/1 -> Gain/1
  Gain1/1 -> Unit Delay/1, Out1/1
  Sum/1 -> Gain1/1
  Gain/1 -> Sum/2

== matlab function Modelo_DINAMICO_2021/Non-linear 6 DOF model/MATLAB Function2 ==
  data: airgaps input; u_1 input; u output; pod parameter; beta parameter
function u  = ag2pos(airgaps, u_1, pod, beta)
% Computes the position and attitute od the pod as a function of the airgaps 
% ═════════════════════════════════════════════════════════════════════════
% Last updated: 27.01.2022
% ═════════════════════════════════════════════════════════════════════════
% INPUT:
%   airgaps   = Vector with airgaps in [m]. The 6 first values correspond
%               to the levitation units, and the 4 last values correspond 
%               to guidance. 
%               Size 10 x 1
%   beta      = Measure acceptance tolerance [-]
%               Scalar
%   pod       = Struct containing data about
%                   *mass (Mass and inertia)
%                   *brakes (Pressures, friction coefficients and forces)
%                   *levitation (Maps of forces)
%                   *guiding (Maps of forces)
%                   *propulsion (Force as a function of velocity). 
%                   *geometry (points of application of forces wrt CG)
%                   *general (simulation parameters)
%   u         = DOF vector in (t-1), containing the estimations of the 
%               position in the y and z directions [m] and the 3 rotation 
%               angles [rad]
%               Size 5 x 1
% OUTPUT:
%   u         = DOF vector, containing the estimations of the position in
%               the y and z directions [m] and the 3 rotation angles [rad]
%               Size 5 x 1
% ═════════════════════════════════════════════════════════════════════════


%%% Input check (4 inputs)
narginchk(4,4);

%%% Ensure inputs are well defined
% airgaps must be a 10 dimensional vector
if ~ismatrix(airgaps) || numel(airgaps) ~= 10
    error('Vector with airgaps is not properly defined');
end

% % Filter incorrect measures
% if any(isnan(airgaps))
%     warning('Signal of unit number %d is incorrect. The system will ignore it, but computation will be slower.', find(isnan(airgaps)));
%     airgaps(isnan(airgaps)) = 0;
% end

% % Beta must be scalar
% if ~(isscalar(beta))
%     error('beta must be an scalar')
% end


%%% Auxiliar vectors initialization 
coder.varsize('y_aux'); 
coder.varsize('z_aux'); 
coder.varsize('rotx_aux');
coder.varsize('roty_aux');
coder.varsize('rotz_aux')
coder.varsize('malfunction'); 

y_aux       = zeros(4,1);
idx_y       = false(4,1);
z_aux       = zeros(6,1);
idx_z       = false(6,1);
rotx_aux    = zeros(3,1);
idxx        = false(3,1);
roty_aux    = zeros(6,1);
idxy        = false(6,1);
rotz_aux    = zeros(2,1);
idxz        = false(2,1);
malfunction = true(11,1);
y = 0; z = 0; rotx = 0; roty = 0; rotz = 0;

%%% Attitude
rotx_aux(1) = asin((airgaps(1) - airgaps(4))/(2 * pod.geometry.y_LEV));
rotx_aux(2) = asin((airgaps(2) - airgaps(5))/(2 * pod.geometry.y_LEV));
rotx_aux(3) = asin((airgaps(3) - airgaps(6))/(2 * pod.geometry.y_LEV));

roty_aux(1) = asin((airgaps(5) - airgaps(4))/(    pod.geometry.z_LEV));
roty_aux(2) = asin((airgaps(6) - airgaps(4))/(2 * pod.geometry.z_LEV));
roty_aux(3) = asin((airgaps(6) - airgaps(5))/(    pod.geometry.z_LEV));
roty_aux(4) = asin((airgaps(3) - airgaps(2))/(    pod.geometry.z_LEV));
roty_aux(5) = asin((airgaps(3) - airgaps(1))/(2 * pod.geometry.z_LEV));
roty_aux(6) = asin((airgaps(2) - airgaps(1))/(    pod.geometry.z_LEV));

rotz_aux(1) = asin((airgaps(8) - airgaps(7 ))/(pod.geometry.x_G_front + pod.geometry.x_G_rear));
rotz_aux(1) = asin((airgaps(9) - airgaps(10))/(pod.geometry.x_G_front + pod.geometry.x_G_rear));

while any(malfunction)
    rotx = mean(rotx_aux);
    roty = mean(roty_aux);
    rotz = mean(rotz_aux);

    resx = abs(rotx_aux - rotx);
    resy = abs(roty_aux - roty);
    resz = abs(rotz_aux - rotz);

    idxx =  (resx> abs(beta*rotx));
    idxy =  (resy> abs(beta*roty));
    idxz =  (resz> abs(beta*rotz));

    malfunction = [idxx; idxy; idxz];

    rotx_aux = rotx_aux(~(idxx));
    roty_aux = roty_aux(~(idxy));
    rotz_aux = rotz_aux(~(idxz));
end

malfunction = true(10,1);

%%% Position
x_G     = 0.5 * (pod.geometry.x_G_front + pod.geometry.x_G_rear);
x_LEV   = 0.5 * (pod.geometry.x_LEV_front + pod.geometry.x_LEV_rear);

y_aux(1) = airgaps(7)    + pod.geometry.y_G * cos(rotz) +   x_G * sin(rotz);
y_aux(2) = airgaps(8)    + pod.geometry.y_G * cos(rotz) -   x_G * sin(rotz);
y_aux(3) = - airgaps(9)  - pod.geometry.y_G * cos(rotz) - x_G * sin(rotz);
y_aux(4) = - airgaps(10) - pod.geometry.y_G * cos(rotz) + x_G * sin(rotz);

z_aux(1) = airgaps(1)  + pod.geometry.z_LEV * cos(roty) + x_LEV * sin(roty) - pod.geometry.y_LEV * sin(rotx);
z_aux(2) = airgaps(2)  + pod.geometry.z_LEV * cos(roty)                     - pod.geometry.y_LEV * sin(rotx);
z_aux(3) = airgaps(3)  + pod.geometry.z_LEV * cos(roty) - x_LEV * sin(roty) - pod.geometry.y_LEV * sin(rotx);
z_aux(4) = airgaps(4)  + pod.geometry.z_LEV * cos(roty) + x_LEV * sin(roty) + pod.geometry.y_LEV * sin(rotx);
z_aux(5) = airgaps(5)  + pod.geometry.z_LEV * cos(roty)                     + pod.geometry.y_LEV * sin(rotx);
z_aux(6) = airgaps(6)  + pod.geometry.z_LEV * cos(roty) - x_LEV * sin(roty) + pod.geometry.y_LEV * sin(rotx);


while any(malfunction)
    y = mean(y_aux);
    z = mean(z_aux);

    resy = abs(y_aux - y);
    resz = abs(z_aux - z);

    idx_y = (resy>beta*y);
    idx_z = (resz>beta*z);

    malfunction = [idxy; idxz];

    y_aux = y_aux(~(idx_y));
    z_aux = z_aux(~(idx_z));
end

u = [y, z, rotx, roty, rotz]';

u(isnan(u)) = u_1(isnan(u));

end

== matlab function Modelo_DINAMICO_2021/Non-linear 6 DOF model/H7 Pod Dynamic model/Levitation/MATLAB Function ==
  data: v input; F output; pod parameter
function F = HEMSdrag(v, pod)
% Computes the drag force (N) of one HEMS unit as a function of the 
% velocity (m/s)
% ═════════════════════════════════════════════════════════════════════════
% Last updated: 15.12.2021
% ═════════════════════════════════════════════════════════════════════════

F = pod.levitation.drag_1_unit.poly.p3*v^3 + ...
    pod.levitation.drag_1_unit.poly.p2*v^2 + ...
    pod.levitation.drag_1_unit.poly.p1*v   ;

== matlab function Modelo_DINAMICO_2021/Non-linear 6 DOF model/H7 Pod Dynamic model/Guidance/MATLAB Function ==
  data: v input; F output
function F = EMSdrag(v)
% Computes the drag force (N) of one EMS units as a function of 
% its velocity (m/s)
% ═════════════════════════════════════════════════════════════════════════
% Last updated: 15.12.2021
% ════════════════════════════════════════════════════════════════════════

F = 0;

== matlab function Modelo_DINAMICO_2021/Non-linear 6 DOF model/H7 Pod Dynamic model/Guidance/MATLAB Function1 ==
  data: airgap input; F output; intensity input; pod parameter
function F = EMSlev(airgap, intensity, pod)
% Computes the levitation force (N) of all the EMS units as a function of 
% their air gaps (mm) and intensities (A)
% ═════════════════════════════════════════════════════════════════════════
% Last updated: 24.03.2022
% ════════════════════════════════════════════════════════════════════════

x   = airgap(7:10);
y   = intensity(7:10);

F = pod.guiding.poly.p00 + ...
    pod.guiding.poly.p10.*x + ...
    pod.guiding.poly.p01.*y + ...
    pod.guiding.poly.p20.*x.^2 + ...
    pod.guiding.poly.p11.*x.*y + ...
    pod.guiding.poly.p02.*y.^2 + ...
    pod.guiding.poly.p21.*x.^2.*y + ...
    pod.guiding.poly.p12.*x.*y.^2 + ...
    pod.guiding.poly.p03.*y.^3 + ...
    pod.guiding.poly.p22.*x.^2.*y.^2 + ...
    pod.guiding.poly.p13.*x.*y.^3 + ...
    pod.guiding.poly.p04.*y.^4 + ...
    pod.guiding.poly.p23.*x.^2.*y.^3 + ...
    pod.guiding.poly.p14.*x.*y.^4 + ...
    pod.guiding.poly.p05.*y.^5;

== matlab function Modelo_DINAMICO_2021/Non-linear 6 DOF model/H7 Pod Dynamic model/LIM/MATLAB Function ==
  data: v input; acceleration_flag input; F output; pod parameter
function F = LIMtraction(v, acceleration_flag, pod)
% Computes the traction force (N) of the LIM as a function of 
% the absolute velocity of the prototype (m/s)
% ═════════════════════════════════════════════════════════════════════════
% Last updated: 20.12.2021
% ═════════════════════════════════════════════════════════════════════════

if acceleration_flag == 1
    F = pod.propulsion.poly.p3*v^3 + ...
        pod.propulsion.poly.p2*v^2 + ...
        pod.propulsion.poly.p1*v   + ...
        pod.propulsion.poly.p0;

else
    F = pod.propulsion.br_poly.p2*v^2 + ...
        pod.propulsion.br_poly.p1*v   + ...
        pod.propulsion.br_poly.p0;
end

== matlab function Modelo_DINAMICO_2021/Non-linear 6 DOF model/H7 Pod Dynamic model/LIM/MATLAB Function1 ==
  data: v input; x input; sign output; pod parameter
function sign = LIMdirection(v, x, pod)
% Decides if the LIM force is being applied to accelerate or to brake 
% by comparing the position of the pod with a predefined treshold
% ═════════════════════════════════════════════════════════════════════════
% Last updated: 20.12.2021
% ═════════════════════════════════════════════════════════════════════════

if x >= pod.brakes.d && v > 0    
    sign = -1;
elseif x >= pod.brakes.d && v <= 0
    sign = 0;
else
    sign = 1;
end

== matlab function Modelo_DINAMICO_2021/Non-linear 6 DOF model/H7 Pod Dynamic model/Levitation/MATLAB Function1 ==
  data: airgap input; F output; intensity input; pod parameter
function F = HEMSlev(airgap, intensity, pod)
% Computes the levitation force (N) of all the HEMS units as a function of 
% their air gaps (mm) and intensities (A)
% ═════════════════════════════════════════════════════════════════════════
% Last updated: 15.12.2021
% ════════════════════════════════════════════════════════════════════════

x   = airgap(1:6);
y   = intensity(1:6);

F = pod.levitation.poly_1_unit.p00 + ...
    pod.levitation.poly_1_unit.p10.*x + ...
    pod.levitation.poly_1_unit.p01.*y + ...
    pod.levitation.poly_1_unit.p20.*x.^2 + ...
    pod.levitation.poly_1_unit.p11.*x.*y + ...
    pod.levitation.poly_1_unit.p02.*y.^2 + ...
    pod.levitation.poly_1_unit.p21.*x.^2.*y + ...
    pod.levitation.poly_1_unit.p12.*x.*y.^2 + ...
    pod.levitation.poly_1_unit.p03.*y.^3;

== matlab function Modelo_DINAMICO_2021/Non-linear 6 DOF model/H7 Pod Dynamic model/MATLAB Function ==
  data: F input; F_e output; attitude input; pod parameter
function F_e = BF2E(F, attitude, pod)
% Computes the total force in absoute axis
% ═════════════════════════════════════════════════════════════════════════
% Last updated: 27.12.2021
% ═════════════════════════════════════════════════════════════════════════
F     = reshape(F, [3 1]);


F_e = attitude * F + pod.mass.mass * [0 0 9.81]';

== matlab function Modelo_DINAMICO_2021/Non-linear 6 DOF model/H7 Pod Dynamic model/Wheels/MATLAB Function ==
  data: z input; F output; pod parameter; z_CF output
function [F, z_CF] = rollingFriction(z, pod)
% Computes the rolling resistance force (N) of the wheels. It distinguishes
% 3 cases: 
%   (1) z = 0. Pod touching the ground
%   (2) z = z_max. Pod touching the ceiling. It is assumed no current
%   applied to the HEMS. 
%   (3) Otherwise. Pod levitating. 
% ═════════════════════════════════════════════════════════════════════════
% Last updated: 26.12.2021
% ═════════════════════════════════════════════════════════════════════════

% F_LEV worst case scenario computation
x   = 12; % [mm]
y   = 0;  % [A]

F_LEV = pod.levitation.poly_1_unit.p00 + ...
        pod.levitation.poly_1_unit.p10.*x + ...
        pod.levitation.poly_1_unit.p01.*y + ...
        pod.levitation.poly_1_unit.p20.*x.^2 + ...
        pod.levitation.poly_1_unit.p11.*x.*y + ...
        pod.levitation.poly_1_unit.p02.*y.^2 + ...
        pod.levitation.poly_1_unit.p21.*x.^2.*y + ...
        pod.levitation.poly_1_unit.p12.*x.*y.^2 + ...
        pod.levitation.poly_1_unit.p03.*y.^3;

% Main algorithm
if z == 0
    F_N   = pod.mass.mass * 9.81;
    z_CF  = - pod.geometry.z_CF;
elseif z == pod.general.z_range
    F_N   = 6 * F_LEV - pod.mass.mass * 9.81;
    z_CF  = pod.geometry.z_CF;
else
    F_N   = 0;
    z_CF  = 0;
end

F = pod.wheels.number * pod.wheels.roll_coef * F_N;

== matlab function Modelo_DINAMICO_2021/Non-linear 6 DOF model/H7 Pod Dynamic model/Brakes/MATLAB Function ==
  data: x input; velocity input; F output; emergency input; F_N output; pod parameter
function [F, F_N] = brakes_activation(x, velocity, emergency, pod)
% Computes the braking force of the pneumatic actuators if and only if 
%     (1) The emergency flag has been raised
%     (2) The pod is above the acceleration phase distance
% ═════════════════════════════════════════════════════════════════════════
% Last updated: 20.12.2021
% ═════════════════════════════════════════════════════════════════════════

if (emergency == 1 && x >= pod.brakes.d && velocity >= 0)
    F       = pod.brakes.force * ones(pod.brakes.n,1);
    F_N     = pod.brakes.normal_force * ones(pod.brakes.n,1);
else
    F       = zeros(pod.brakes.n,1);
    F_N     = zeros(pod.brakes.n,1);
end

== matlab function Modelo_DINAMICO_2021/Non-linear 6 DOF model/MATLAB Function ==
  data: r input; y output; rot input; pod parameter
function y = pos2ag3D(r, rot, pod)
% Computes the airgaps as a function of the position and the attitude
% ═════════════════════════════════════════════════════════════════════════
% Last updated: 02.02.2022
% ═════════════════════════════════════════════════════════════════════════

y_CG  = r(1);
z_CG  = r(2);
rot_x = rot(1);
rot_y = rot(2);
rot_z = rot(3); 

AG_0  = 10e-3;

AG_1  = z_CG  -  pod.geometry.z_LEV * cos(rot_y)  -  pod.geometry.x_LEV_front * sin(rot_y)  +  pod.geometry.y_LEV * sin(rot_x);
AG_2  = z_CG  -  pod.geometry.z_LEV * cos(rot_y)                                            +  pod.geometry.y_LEV * sin(rot_x);
AG_3  = z_CG  -  pod.geometry.z_LEV * cos(rot_y)  +  pod.geometry.x_LEV_rear  * sin(rot_y)   +  pod.geometry.y_LEV * sin(rot_x);
AG_4  = z_CG  -  pod.geometry.z_LEV * cos(rot_y)  -  pod.geometry.x_LEV_front * sin(rot_y)  -  pod.geometry.y_LEV * sin(rot_x);
AG_5  = z_CG  -  pod.geometry.z_LEV * cos(rot_y)                                            -  pod.geometry.y_LEV * sin(rot_x);
AG_6  = z_CG  -  pod.geometry.z_LEV * cos(rot_y)  +  pod.geometry.x_LEV_rear  * sin(rot_y)  -  pod.geometry.y_LEV * sin(rot_x);

AG_7  = - y_CG  - pod.geometry.x_G_front * sin(rot_z) + AG_0;
AG_8  = - y_CG  + pod.geometry.x_G_rear  * sin(rot_z) + AG_0;
AG_9  =   y_CG  + pod.geometry.x_G_front * sin(rot_z) + AG_0;
AG_10 =   y_CG  - pod.geometry.x_G_rear  * sin(rot_z) + AG_0;

y = [AG_1; AG_2; AG_3; AG_4; AG_5; AG_6; AG_7; AG_8; AG_9; AG_10];

y(y<0)=0;
